simulink model "cassie"  (R2017b)
settings: Solver=FixedStepAuto  StartTime=0.0  StopTime=inf  RelTol=1e-3
InitFcn:
  | PreFunctions.PreParams
undefined symbols (not defined in the file or in its folder): UserParams
libraries: xpcethercatlib x47, ComponentLibrary x10, slrtlib x5, xpcutilitieslib x2, xpcrtudplib x2, dsparch4 x2
(part 2 of 2)

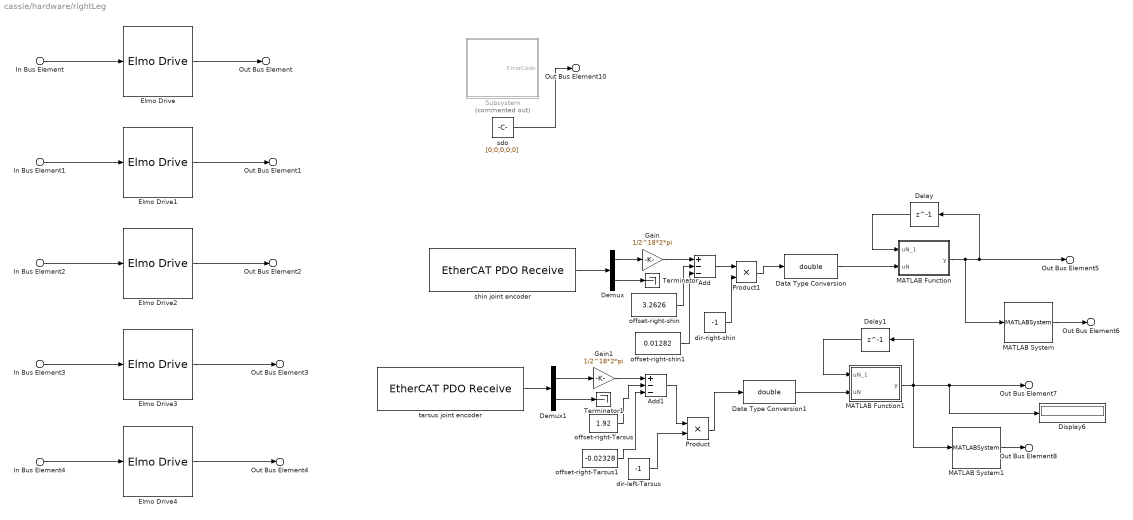
== system cassie/hardware/rightLeg ==
  In Bus Element4 : Inport  PortName=InBus  Element=footDrive
  In Bus Element : Inport  PortName=InBus  Element=hipRollDrive
  In Bus Element1 : Inport  PortName=InBus  Element=hipYawDrive
  In Bus Element2 : Inport  PortName=InBus  Element=hipPitchDrive
  In Bus Element3 : Inport  PortName=InBus  Element=kneeDrive
  Add : Sum  Inputs=+--
  Add1 : Sum  Inputs=+--
  Data Type Conversion : DataTypeConversion  OutDataTypeStr=double
  Data Type Conversion1 : DataTypeConversion  OutDataTypeStr=double
  Delay : Delay  DelayLength=1
  Delay1 : Delay  DelayLength=1
  Demux : Demux  Outputs=2
  Demux1 : Demux  Outputs=2
  Display6 : Display
  Elmo Drive : ComponentLibrary/RealTime/Elmo Drive  ethercatName=RightHipRoll  slaveAddress=1005  currentLimit=65  gearRatio=1  encoderCounts=2^18  Offset=122004
      link override Control Word PDO Transmit: sig_offset=2144  sample_time=0.001000
      link override Mode of Operation PDO Transmit: sig_offset=2160  sample_time=0.001000
      link override Status Word PDO Receive: sig_offset=2176  sample_time=0.001000
      link override Target Torque PDO Transmit: sig_offset=2128  sample_time=0.001000
  Elmo Drive1 : ComponentLibrary/RealTime/Elmo Drive  ethercatName=RightHipYaw  slaveAddress=1006  currentLimit=11.31  gearRatio=1  encoderCounts=2^19  Offset=284898
      link override Mode of Operation PDO Transmit: sig_name=RightHipYaw.Outputs.Modes of operation  sig_offset=1544  sig_type=int8  sample_time=0.000500
      link override Position Actual PDO Receive: sample_time=0.0005  sig_offset=2128
      link override Status Word PDO Receive: sample_time=0.000500  sig_offset=2176
      link override Torque Actual PDO Receive: sample_time=0.000500
      link override Velocity Actual PDO Receive: sig_offset=2128  sample_time=0.001000
  Elmo Drive2 : ComponentLibrary/RealTime/Elmo Drive  ethercatName=RightHipPitch  slaveAddress=1007  currentLimit=65  gearRatio=1  encoderCounts=2^20  Offset=679800
      link override Mode of Operation PDO Transmit: sig_name=RightHipPitch.Outputs.Modes of operation  sig_offset=1672  sig_type=int8  sample_time=0.000500
      link override Status Word PDO Receive: sample_time=0.000500
      link override Target Torque PDO Transmit: sample_time=0.000500
  Elmo Drive3 : ComponentLibrary/RealTime/Elmo Drive  ethercatName=RightKnee  slaveAddress=1008  currentLimit=65  gearRatio=1  encoderCounts=2^20  Offset=901342+9462
      link override Mode of Operation PDO Transmit: sig_offset=1800  sample_time=0.0005
  Elmo Drive4 : ComponentLibrary/RealTime/Elmo Drive  ethercatName=RightFoot  slaveAddress=1009  currentLimit=7.07  gearRatio=1  encoderCounts=2^19  Offset=296723
  Gain : Gain  Gain=1/2^18*2*pi  ParamDataTypeStr=double  OutDataTypeStr=double
  Gain1 : Gain  Gain=1/2^18*2*pi  ParamDataTypeStr=double  OutDataTypeStr=double
  MATLAB Function : MATLAB Function  TreatAsAtomicUnit=on
  MATLAB Function1 : MATLAB Function  TreatAsAtomicUnit=on
  MATLAB System : MATLABSystem  System=FilterSystem  a=[1 -1.76575295625865 0.790448801800725]  b=[12.3479227710395 12.3479227710395 -12.3479227710395 -12.3479227710395]  SimulateUsing=Code generation
      mask Type: FilterSystem
      mask Display: disp('Filter');
  MATLAB System1 : MATLABSystem  System=FilterSystem  a=[1 -1.76575295625865 0.790448801800725]  b=[12.3479227710395 12.3479227710395 -12.3479227710395 -12.3479227710395]  SimulateUsing=Code generation
      mask Type: FilterSystem
      mask Display: disp('Filter');
  Product : Product
  Product1 : Product
  Subsystem : Subsystem  Commented=on
  Terminator : Terminator
  Terminator1 : Terminator
  dir-left-Tarsus : Constant  Value=-1
  dir-right-shin : Constant  Value=-1
  offset-right-Tarsus : Constant  Value=1.92
  offset-right-Tarsus1 : Constant  Value=-0.02328
  offset-right-shin : Constant  Value=3.2626
  offset-right-shin1 : Constant  Value=0.01282
  sdo : Constant  Value=[0;0;0;0;0]  OutDataTypeStr=uint16
  shin joint encoder : xpcethercatlib/EtherCAT PDO Receive  Priority=2  sig_name=Term 5 (EL5042).FB Inputs Channel 1.Position  sig_offset=1512  sig_type=uint32  type_size=32  sig_dim=2  device_id=0  sample_time=0.000500
      settings: SourceProductName=Simulink Real-Time  SourceProductBaseCode=XP
  tarsus joint encoder : xpcethercatlib/EtherCAT PDO Receive  Priority=2  sig_name=Term 5 (EL5042).FB Inputs Channel 2.Position  sig_offset=1592  sig_type=uint32  type_size=32  sig_dim=2  device_id=0  sample_time=0.000500
      settings: SourceProductName=Simulink Real-Time  SourceProductBaseCode=XP
  Out Bus Element : Outport  PortName=OutBus  Element=hipRollDrive
  Out Bus Element1 : Outport  PortName=OutBus  Element=hipYawDrive
  Out Bus Element2 : Outport  PortName=OutBus  Element=hipPitchDrive
  Out Bus Element3 : Outport  PortName=OutBus  Element=kneeDrive
  Out Bus Element4 : Outport  PortName=OutBus  Element=footDrive
  Out Bus Element5 : Outport  PortName=OutBus  Element=shinJoint.position
  Out Bus Element6 : Outport  PortName=OutBus  Element=shinJoint.velocity
  Out Bus Element7 : Outport  PortName=OutBus  Element=tarsusJoint.position
  Out Bus Element8 : Outport  PortName=OutBus  Element=tarsusJoint.velocity
  Out Bus Element10 : Outport  PortName=OutBus  Element=ErrorCode
  wires:
  In Bus Element/1 -> Elmo Drive/1
  Elmo Drive/1 -> Out Bus Element/1
  In Bus Element1/1 -> Elmo Drive1/1
  Elmo Drive1/1 -> Out Bus Element1/1
  In Bus Element2/1 -> Elmo Drive2/1
  Elmo Drive2/1 -> Out Bus Element2/1
  In Bus Element3/1 -> Elmo Drive3/1
  Elmo Drive3/1 -> Out Bus Element3/1
  Elmo Drive4/1 -> Out Bus Element4/1
  In Bus Element4/1 -> Elmo Drive4/1
  Product1/1 -> Data Type Conversion/1
  MATLAB System/1 -> Out Bus Element6/1
  MATLAB System1/1 -> Out Bus Element8/1
  shin joint encoder/1 -> Demux/1
  Demux/1 -> Gain/1
  Demux/2 -> Terminator/1
  tarsus joint encoder/1 -> Demux1/1
  Product/1 -> Data Type Conversion1/1
  Demux1/1 -> Gain1/1
  Demux1/2 -> Terminator1/1
  Gain/1 -> Add/1
  offset-right-shin/1 -> Add/2
  offset-right-Tarsus/1 -> Add1/2
  Gain1/1 -> Add1/1
  dir-left-Tarsus/1 -> Product/2
  Add1/1 -> Product/1
  Add/1 -> Product1/1
  dir-right-shin/1 -> Product1/2
  offset-right-shin1/1 -> Add/3
  offset-right-Tarsus1/1 -> Add1/3
  MATLAB Function/1(y) -> MATLAB System/1, Out Bus Element5/1, Delay/1
  Delay/1 -> MATLAB Function/1(uN_1)
  Data Type Conversion/1 -> MATLAB Function/2(uN)
  Data Type Conversion1/1 -> MATLAB Function1/2(uN)
  Delay1/1 -> MATLAB Function1/1(uN_1)
  MATLAB Function1/1(y) -> MATLAB System1/1, Delay1/1, Display6/1, Out Bus Element7/1
  sdo/1 -> Out Bus Element10/1

== system cassie/output/For Each Subsystem ==
  In1 : Inport  Partition=on  PartitionDimension=1  PartitionWidth=1  PartitionOffset=0
  For Each : ForEach  DisableCoverage=on  IndexMode=One-based
  MyButtrtworth1 : dsparch4/Biquad Filter  Tag=BlockMethodSubSystem  IIRFiltStruct=Direct form II  CoeffSource=Specify via dialog  BiQuadCoeffs=[1 2 1 1 -1.99718299857855919 0.99718696075026636]  a0Flag=Warning  IC=0  ICnum=0  ICden=0  InputProcessing=Columns as channels (frame based)  denAccumFracLength=30  denProdOutputFracLength=30  secondMemoryFracLength=15  roundingMode=Floor  overflowMode=off  ScaleValues=[9.90542926808879355e-07;1]  optimizeScaleValues=on  ScaleValueMode=Specify via input port (g)  scaleValueFracLength=14  FilterSource=Specify via dialog  FilterObject=BQF
      settings: SourceProductName=DSP System Toolbox
  Out1 : Outport  ConcatenationDimension=1
  wires:
  In1/1 -> MyButtrtworth1/1
  MyButtrtworth1/1 -> Out1/1

== system cassie/output/For Each Subsystem1 ==
  In1 : Inport  Partition=on  PartitionDimension=1  PartitionWidth=1  PartitionOffset=0
  For Each : ForEach  DisableCoverage=on  IndexMode=One-based
  MyButtrtworth1 : dsparch4/Biquad Filter  Tag=BlockMethodSubSystem  IIRFiltStruct=Direct form II  CoeffSource=Specify via dialog  BiQuadCoeffs=[1 2 1 1 -1.99718299857855919 0.99718696075026636]  a0Flag=Warning  IC=0  ICnum=0  ICden=0  InputProcessing=Columns as channels (frame based)  denAccumFracLength=30  denProdOutputFracLength=30  secondMemoryFracLength=15  roundingMode=Floor  overflowMode=off  ScaleValues=[9.90542926808879355e-07;1]  optimizeScaleValues=on  ScaleValueMode=Specify via input port (g)  scaleValueFracLength=14  FilterSource=Specify via dialog  FilterObject=BQF
      settings: SourceProductName=DSP System Toolbox
  Out1 : Outport  ConcatenationDimension=1
  wires:
  In1/1 -> MyButtrtworth1/1
  MyButtrtworth1/1 -> Out1/1

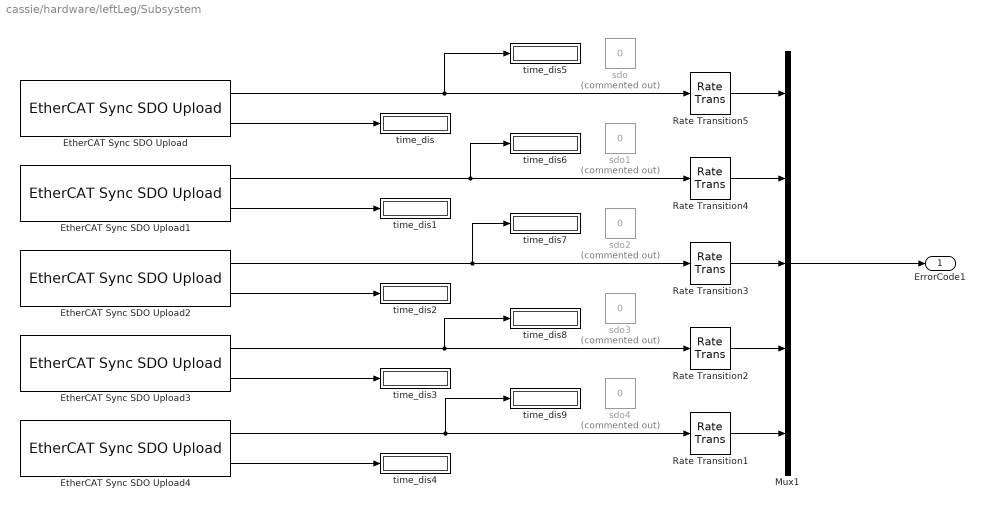
== system cassie/hardware/leftLeg/Subsystem ==
  EtherCAT Sync SDO Upload : xpcethercatlib/EtherCAT Sync SDO Upload  index=24639  subIndex=0  sig_type=uint16  sig_dim=1  device_id=0  slave_name=LeftHipRoll  sample_time=1  slave_addr=1010  selected_slave=Term 1 (EK1100)  timeout=500  slave_found=1
      settings: SourceProductName=Simulink Real-Time  SourceProductBaseCode=XP
  EtherCAT Sync SDO Upload1 : xpcethercatlib/EtherCAT Sync SDO Upload  index=24639  subIndex=0  sig_type=uint16  sig_dim=1  device_id=0  slave_name=LeftHipYaw  sample_time=1  slave_addr=1011  selected_slave=Term 1 (EK1100)  timeout=500  slave_found=1
      settings: SourceProductName=Simulink Real-Time  SourceProductBaseCode=XP
  EtherCAT Sync SDO Upload2 : xpcethercatlib/EtherCAT Sync SDO Upload  index=24639  subIndex=0  sig_type=uint16  sig_dim=1  device_id=0  slave_name=LeftHipPitch  sample_time=1  slave_addr=1012  selected_slave=Term 1 (EK1100)  timeout=500  slave_found=1
      settings: SourceProductName=Simulink Real-Time  SourceProductBaseCode=XP
  EtherCAT Sync SDO Upload3 : xpcethercatlib/EtherCAT Sync SDO Upload  index=24639  subIndex=0  sig_type=uint16  sig_dim=1  device_id=0  slave_name=LeftKnee  sample_time=1  slave_addr=1013  selected_slave=Term 1 (EK1100)  timeout=500  slave_found=1
      settings: SourceProductName=Simulink Real-Time  SourceProductBaseCode=XP
  EtherCAT Sync SDO Upload4 : xpcethercatlib/EtherCAT Sync SDO Upload  index=24639  subIndex=0  sig_type=uint16  sig_dim=1  device_id=0  slave_name=LeftFoot  sample_time=1  slave_addr=1014  selected_slave=Term 1 (EK1100)  timeout=500  slave_found=1
      settings: SourceProductName=Simulink Real-Time  SourceProductBaseCode=XP
  Mux1 : Mux  Inputs=5
  Rate Transition{1..5} (5 alike) : RateTransition  Integrity=off  OutPortSampleTimeMultiple=0.0005
  sdo{,1..4} (5 alike) : Constant  Commented=on  Value=0  OutDataTypeStr=uint16
  time_dis{,1..9} (10 alike) : Display
  ErrorCode1 : Outport
  wires:
  Rate Transition4/1 -> Mux1/2
  Rate Transition5/1 -> Mux1/1
  Rate Transition3/1 -> Mux1/3
  Rate Transition2/1 -> Mux1/4
  EtherCAT Sync SDO Upload4/2 -> time_dis4/1
  EtherCAT Sync SDO Upload2/2 -> time_dis2/1
  EtherCAT Sync SDO Upload4/1 -> Rate Transition1/1, time_dis9/1
  EtherCAT Sync SDO Upload3/1 -> Rate Transition2/1, time_dis8/1
  Rate Transition1/1 -> Mux1/5
  EtherCAT Sync SDO Upload/1 -> Rate Transition5/1, time_dis5/1
  EtherCAT Sync SDO Upload2/1 -> Rate Transition3/1, time_dis7/1
  EtherCAT Sync SDO Upload1/2 -> time_dis1/1
  Mux1/1 -> ErrorCode1/1
  EtherCAT Sync SDO Upload3/2 -> time_dis3/1
  EtherCAT Sync SDO Upload/2 -> time_dis/1
  EtherCAT Sync SDO Upload1/1 -> Rate Transition4/1, time_dis6/1

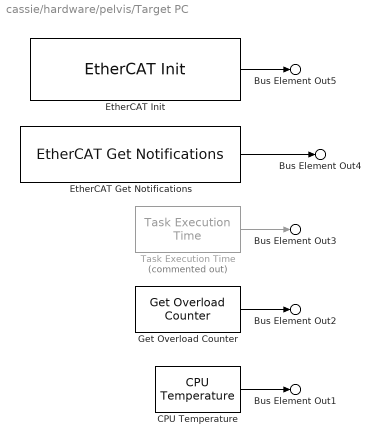
== system cassie/hardware/pelvis/Target PC ==
  CPU Temperature : slrtlib/Target Management/Target Information/CPU Temperature  ts=UserParams.SampleTime
      settings: SourceProductName=Simulink Real-Time  SourceProductBaseCode=XP
  EtherCAT Get Notifications : xpcethercatlib/EtherCAT Get Notifications   device_id=0  sample_time=UserParams.SampleTime
      settings: SourceProductName=Simulink Real-Time  SourceProductBaseCode=XP
  EtherCAT Init : xpcethercatlib/EtherCAT Init   Priority=0  config_file=C:\Users\Robot\Desktop\Casia_biped\Controllers\cassie\xml\robot20220509.xml  device_id=0  pci_bus=pci_bus  pci_slot=pci_slot  pci_function=pci_function  dctuning=0  enaDebug=off  enaDC=on  errLink=on  masterDbg=on  stateChgDbg=off  baseClock=off  masterCfg=off  logFile='c:\dbglog.txt'  sample_time=0.000500  DCMode=2
      settings: SourceProductName=Simulink Real-Time  SourceProductBaseCode=XP
  Get Overload Counter : slrtlib/Target Management/Execution Parameters/Get Overload Counter   ts=UserParams.SampleTime
      settings: SourceProductName=Simulink Real-Time  SourceProductBaseCode=XP
  "Task Execution Time " : slrtlib/Target Management/Execution Parameters/Task Execution Time   Commented=on  ts=UserParams.SampleTime
      settings: SourceProductName=Simulink Real-Time  SourceProductBaseCode=XP
  Bus Element Out5 : Outport  PortName=OutBus  Element=etherCatStatus
  Bus Element Out4 : Outport  PortName=OutBus  Element=etherCatNotifications
  Bus Element Out3 : Outport  PortName=OutBus  Element=taskExecutionTime
  Bus Element Out2 : Outport  PortName=OutBus  Element=overloadCounter
  Bus Element Out1 : Outport  PortName=OutBus  Element=cpuTemperature
  wires:
  Get Overload Counter/1 -> Bus Element Out2/1
  EtherCAT Init/1 -> Bus Element Out5/1
  EtherCAT Get Notifications/1 -> Bus Element Out4/1
  "Task Execution Time "/1 -> Bus Element Out3/1
  CPU Temperature/1 -> Bus Element Out1/1

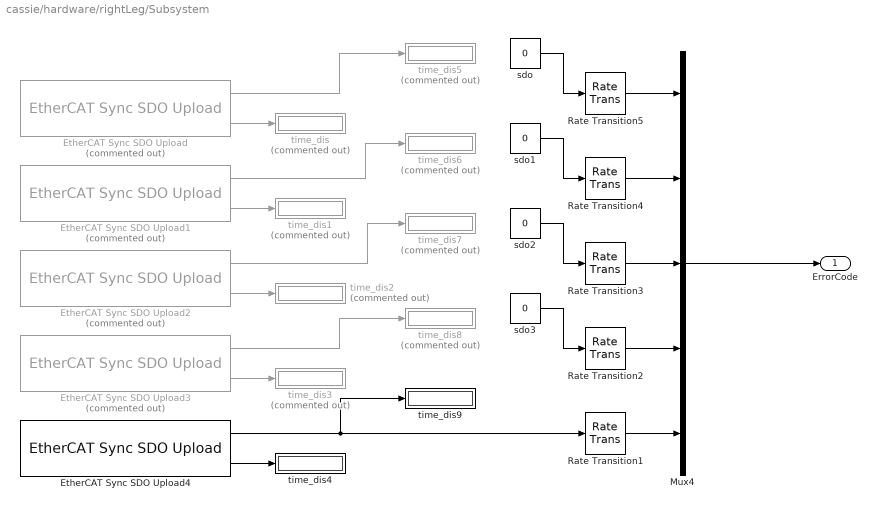
== system cassie/hardware/rightLeg/Subsystem ==
  EtherCAT Sync SDO Upload : xpcethercatlib/EtherCAT Sync SDO Upload  Commented=on  index=24639  subIndex=0  sig_type=uint16  sig_dim=1  device_id=0  slave_name=RightHipRoll  sample_time=1  slave_addr=1005  selected_slave=Term 1 (EK1100)  timeout=500  slave_found=1
      settings: SourceProductName=Simulink Real-Time  SourceProductBaseCode=XP
  EtherCAT Sync SDO Upload1 : xpcethercatlib/EtherCAT Sync SDO Upload  Commented=on  index=24639  subIndex=0  sig_type=uint16  sig_dim=1  device_id=0  slave_name=RightHipYaw  sample_time=1  slave_addr=1006  selected_slave=Term 1 (EK1100)  timeout=500  slave_found=1
      settings: SourceProductName=Simulink Real-Time  SourceProductBaseCode=XP
  EtherCAT Sync SDO Upload2 : xpcethercatlib/EtherCAT Sync SDO Upload  Commented=on  index=24639  subIndex=0  sig_type=uint16  sig_dim=1  device_id=0  slave_name=RightHipPitch  sample_time=1  slave_addr=1007  selected_slave=Term 1 (EK1100)  timeout=500  slave_found=1
      settings: SourceProductName=Simulink Real-Time  SourceProductBaseCode=XP
  EtherCAT Sync SDO Upload3 : xpcethercatlib/EtherCAT Sync SDO Upload  Commented=on  index=24639  subIndex=0  sig_type=uint16  sig_dim=1  device_id=0  slave_name=RightKnee  sample_time=1  slave_addr=1008  selected_slave=Term 1 (EK1100)  timeout=500  slave_found=1
      settings: SourceProductName=Simulink Real-Time  SourceProductBaseCode=XP
  EtherCAT Sync SDO Upload4 : xpcethercatlib/EtherCAT Sync SDO Upload  index=24639  subIndex=0  sig_type=uint16  sig_dim=1  device_id=0  slave_name=RightFoot  sample_time=1  slave_addr=1009  selected_slave=Term 1 (EK1100)  timeout=500  slave_found=1
      settings: SourceProductName=Simulink Real-Time  SourceProductBaseCode=XP
  Mux4 : Mux  Inputs=5
  Rate Transition{1..5} (5 alike) : RateTransition  Integrity=off  OutPortSampleTimeMultiple=0.0005
  sdo{,1..3} (4 alike) : Constant  Value=0  OutDataTypeStr=uint16
  time_dis{,1..3,5..8} (8 alike) : Display  Commented=on
  time_dis4 : Display
  time_dis9 : Display
  ErrorCode : Outport
  wires:
  EtherCAT Sync SDO Upload/2 -> time_dis/1
  EtherCAT Sync SDO Upload1/2 -> time_dis1/1
  EtherCAT Sync SDO Upload2/2 -> time_dis2/1
  EtherCAT Sync SDO Upload3/2 -> time_dis3/1
  EtherCAT Sync SDO Upload4/2 -> time_dis4/1
  EtherCAT Sync SDO Upload1/1 -> time_dis6/1
  EtherCAT Sync SDO Upload2/1 -> time_dis7/1
  EtherCAT Sync SDO Upload3/1 -> time_dis8/1
  EtherCAT Sync SDO Upload4/1 -> Rate Transition1/1, time_dis9/1
  EtherCAT Sync SDO Upload/1 -> time_dis5/1
  Mux4/1 -> ErrorCode/1
  Rate Transition1/1 -> Mux4/5
  Rate Transition2/1 -> Mux4/4
  Rate Transition3/1 -> Mux4/3
  Rate Transition4/1 -> Mux4/2
  Rate Transition5/1 -> Mux4/1
  sdo/1 -> Rate Transition5/1
  sdo1/1 -> Rate Transition4/1
  sdo2/1 -> Rate Transition3/1
  sdo3/1 -> Rate Transition2/1

== matlab function cassie/hardware/leftLeg/MATLAB Function1 ==
  data: uN_1 input; uN input; y output
function y = fcn(uN_1,uN)
    if abs(uN_1 - uN) < 0.5
        y = uN;
    else
       y = uN_1; 
    end

== matlab function cassie/hardware/rightLeg/MATLAB Function ==
  data: uN_1 input; uN input; y output
function y = fcn(uN_1,uN)
    if abs(uN_1 - uN) < 0.5
        y = uN;
    else
       y = uN_1; 
    end

== matlab function cassie/hardware/rightLeg/MATLAB Function1 ==
  data: uN_1 input; uN input; y output
function y = fcn(uN_1,uN)
    if abs(uN_1 - uN) < 0.5
        y = uN;
    else
       y = uN_1; 
    end

== matlab function cassie/hardware/leftLeg/MATLAB Function2 ==
  data: uN_1 input; uN input; y output
function y = fcn(uN_1,uN)
    if abs(uN_1 - uN) < 0.5
        y = uN;
    else
       y = uN_1; 
    end
